simulink model "EMR_vehicle_model"  (R2023a)
settings: Solver=VariableStepAuto  StartTime=0.0  StopTime=10.0  RelTol=1e-3
values from neighbouring files (symbols this model uses):
  A_f = 2    [parameter_definiciton.m]
  air_dens = 1.22521    [parameter_definiciton.m]
  angle_road = atan(slope_road/100)    [parameter_definiciton.m]
  C_d = 0.35    [parameter_definiciton.m]
  f_r = 0.017    [parameter_definiciton.m]
  g = 9.8    [parameter_definiciton.m]
  m_v = 1000    [parameter_definiciton.m]
  wind_speed = 0    [parameter_definiciton.m]
libraries: simulink x1
settings Model: Creator=citcea  LastModifiedBy=citcea

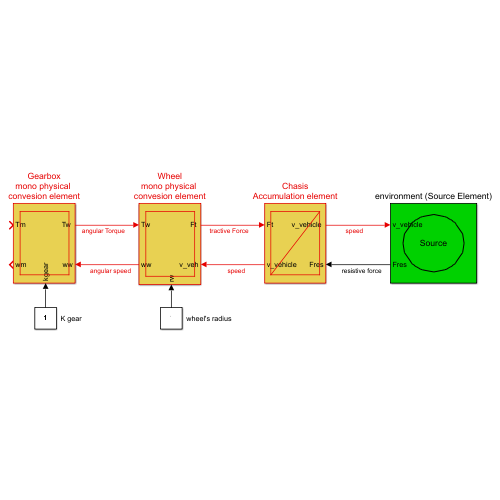
[thumbnail: Simulink's stored preview of the top-level diagram]
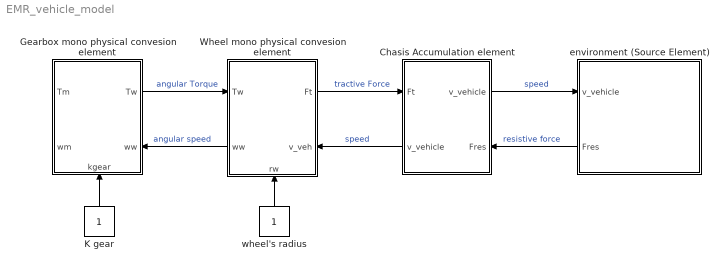
== system EMR_vehicle_model ==
  Chasis Accumulation element : Subsystem  mask(CM){}
      settings: LibrarySourceBlock=simulink/REM/EA  PortSchema="{\"entries\":[{\"content\":{\"sides\":[{\"content\":{\"connectorIds\":[\"In1\",\"Out2\"]},\"type\":\"ConnectorPlacement.EquallySpacedRectSide\",\"uuid\":\"dba36025-b2f5-41cb-9761-d1287a9766e1\"},{\"content\":{\"connectorIds\":[\"Out1\",\"In2\"],\"side\":\"RIGHT\"},\"type\":\"ConnectorPlacement.EquallySpacedRectSide\",\"uuid\":\"3ae5e504-7b8f-4c00-bc0d-c89eccd87070\"},{\"content\":{\"side\":\"TOP\"},\"type\":\"ConnectorPlacement.EquallySpacedRectSide\",\"uuid\":\"a4c04bb5-f94e-4b5c-882d-2c32a11c6b0c\"}]},\"type\":\"ConnectorPlacement.EquallySpacedConnector\",\"uuid\":\"0c2b765b-f129-495b-87a6-76b6e14d78ec\"}],\"packageUris\":[\"http://schema.mathworks.com/mf0/Connector/R2020b\"],\"version\":\"1.0\"}"
      mask Display: plot(0,0,100,100,[10,10,90,90,10],[90,10,10,90,90], [10,90],[10,90])
  Gearbox mono physical convesion element : Subsystem  mask(Hacheur){}
      settings: LibrarySourceBlock=simulink/REM/EC Elec  PortSchema="{\"entries\":[{\"content\":{\"sides\":[{\"content\":{\"connectorIds\":[\"In1\",\"Out2\"]},\"type\":\"ConnectorPlacement.EquallySpacedRectSide\",\"uuid\":\"add9fadb-0fb4-43ab-a2d0-7727804eb2c0\"},{\"content\":{\"connectorIds\":[\"Out1\",\"In3\"],\"side\":\"RIGHT\"},\"type\":\"ConnectorPlacement.EquallySpacedRectSide\",\"uuid\":\"87b3f5c0-7da9-421a-ae8a-66afee038ab7\"},{\"content\":{\"side\":\"TOP\"},\"type\":\"ConnectorPlacement.EquallySpacedRectSide\",\"uuid\":\"1a4f8f42-25ac-452e-8ff7-6a9f16bc9892\"},{\"content\":{\"connectorIds\":[\"In2\"],\"side\":\"BOTTOM\"},\"type\":\"ConnectorPlacement.EquallySpacedRectSide\",\"uuid\":\"62447f74-8a92-4f32-9436-8aa69c6390a6\"}]},\"type\":\"ConnectorPlacement.EquallySpacedConnector\",\"uuid\":\"bc965109-6171-440e-b0fd-d7c986fb98ff\"}],\"packageUris\":[\"http://schema.mathworks.com/mf0/Connector/R2020b\"],\"version\":\"1.0\"}"
      mask Display: plot(0,0,100,100,[10,10,90,90,10],[90,10,10,90,90])
  K gear : Constant
  Wheel mono physical convesion element : Subsystem  mask(Hacheur){}
      settings: LibrarySourceBlock=simulink/REM/EC Elec  PortSchema="{\"entries\":[{\"content\":{\"sides\":[{\"content\":{\"connectorIds\":[\"In1\",\"Out2\"]},\"type\":\"ConnectorPlacement.EquallySpacedRectSide\",\"uuid\":\"add9fadb-0fb4-43ab-a2d0-7727804eb2c0\"},{\"content\":{\"connectorIds\":[\"Out1\",\"In3\"],\"side\":\"RIGHT\"},\"type\":\"ConnectorPlacement.EquallySpacedRectSide\",\"uuid\":\"87b3f5c0-7da9-421a-ae8a-66afee038ab7\"},{\"content\":{\"side\":\"TOP\"},\"type\":\"ConnectorPlacement.EquallySpacedRectSide\",\"uuid\":\"1a4f8f42-25ac-452e-8ff7-6a9f16bc9892\"},{\"content\":{\"connectorIds\":[\"In2\"],\"side\":\"BOTTOM\"},\"type\":\"ConnectorPlacement.EquallySpacedRectSide\",\"uuid\":\"cb138da9-d7db-4398-93fc-4ebc55a3031f\"}]},\"type\":\"ConnectorPlacement.EquallySpacedConnector\",\"uuid\":\"bc965109-6171-440e-b0fd-d7c986fb98ff\"}],\"packageUris\":[\"http://schema.mathworks.com/mf0/Connector/R2020b\"],\"version\":\"1.0\"}"
      mask Display: plot(0,0,100,100,[10,10,90,90,10],[90,10,10,90,90])
  environment (Source Element) : Subsystem
      settings: LibrarySourceBlock=simulink/REM/SE  PortSchema="{\"entries\":[{\"content\":{\"sides\":[{\"content\":{\"connectorIds\":[\"In1\",\"Out1\"]},\"type\":\"ConnectorPlacement.EquallySpacedRectSide\",\"uuid\":\"5172ac9f-d5c1-4cd8-b96a-59474b42a5b1\"},{\"content\":{\"side\":\"RIGHT\"},\"type\":\"ConnectorPlacement.EquallySpacedRectSide\",\"uuid\":\"2f1e5561-012a-4a4f-9618-a2ea7815b4bb\"},{\"content\":{\"side\":\"TOP\"},\"type\":\"ConnectorPlacement.EquallySpacedRectSide\",\"uuid\":\"04863bbd-e2a6-484f-917f-c8a12d5dbdba\"}]},\"type\":\"ConnectorPlacement.EquallySpacedConnector\",\"uuid\":\"d1a021b9-616a-4321-9b00-fb5e0223e97f\"}],\"packageUris\":[\"http://schema.mathworks.com/mf0/Connector/R2020b\"],\"version\":\"1.0\"}"
      mask Display:
      | plot(0,0,100,100, 1.2*[50,57.68,60.77,63.08,64.97,66.58,68,69.26,70.4, 	71.42,72.36,78.28,80,78.28,72.36,71.42,70.4, 	69.26,68,66.58,64.97,63.08,60.77,57.68,50,42.32, 	39.23,36.92,35.03,33.42,32,30.74,29.6,28.58, 	27.64,21.72,20,21.72,27.64,28.58,29.6,30.74,32, 	33.42,35.03,36.92,39.23,42.32,50]-10, 1.2*[20,21,22,23,24,25,26,27,28,29,30,40,50,60,70,71,72, 	73,74,75,76,77,78,79,80,79,78,77,76,75,74,73,72, 	71,70,60,50,40,30,29,28,27,26,25,24,23,22,21,20]-10)
      | disp('Source')
  wheel's radius : Constant
  wires:
  Chasis Accumulation element/1("v_vehicle ") -> environment (Source Element)/1(v_vehicle)  "speed"
  environment (Source Element)/1(Fres) -> Chasis Accumulation element/2(Fres)  "resistive force"
  Wheel mono physical convesion element/1("Ft ") -> Chasis Accumulation element/1(Ft)  "tractive Force"
  Chasis Accumulation element/2(v_vehicle) -> Wheel mono physical convesion element/3(v_veh)  "speed"
  wheel's radius/1 -> Wheel mono physical convesion element/2(rw)
  Gearbox mono physical convesion element/1("Tw ") -> Wheel mono physical convesion element/1(Tw)  "angular Torque"
  Wheel mono physical convesion element/2(ww) -> Gearbox mono physical convesion element/3(ww)  "angular speed"
  K gear/1 -> Gearbox mono physical convesion element/2(kgear)

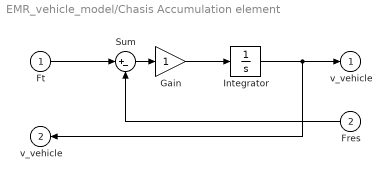
== system EMR_vehicle_model/Chasis Accumulation element ==
  Ft : Inport
  Fres : Inport  Port=2
  Gain : Gain
  Integrator : Integrator
  Sum : Sum  Inputs=|+-
  "v_vehicle " : Outport  InitialOutput=0
  v_vehicle : Outport  Port=2  InitialOutput=0
  wires:
  Gain/1 -> Integrator/1
  Sum/1 -> Gain/1
  Integrator/1 -> v_vehicle/1, "v_vehicle "/1
  Ft/1 -> Sum/1
  Fres/1 -> Sum/2

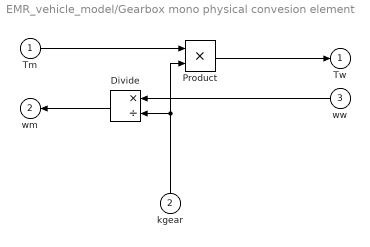
== system EMR_vehicle_model/Gearbox mono physical convesion element ==
  Tm : Inport
  kgear : Inport  Port=2
  ww : Inport  Port=3
  Divide : Product  Inputs=*/
  Product : Product
  "Tw " : Outport  InitialOutput=0
  wm : Outport  Port=2  InitialOutput=0
  wires:
  Divide/1 -> wm/1
  kgear/1 -> Divide/2, Product/2
  ww/1 -> Divide/1
  Product/1 -> "Tw "/1
  Tm/1 -> Product/1

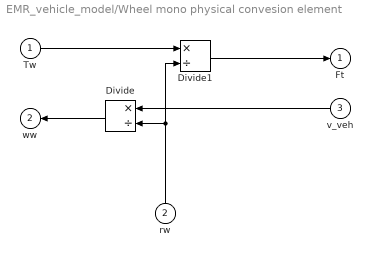
== system EMR_vehicle_model/Wheel mono physical convesion element ==
  Tw : Inport
  rw : Inport  Port=2
  v_veh : Inport  Port=3
  Divide : Product  Inputs=*/
  Divide1 : Product  Inputs=*/
  "Ft " : Outport  InitialOutput=0
  ww : Outport  Port=2  InitialOutput=0
  wires:
  Divide/1 -> ww/1
  v_veh/1 -> Divide/1
  rw/1 -> Divide1/2, Divide/2
  Divide1/1 -> "Ft "/1
  Tw/1 -> Divide1/1

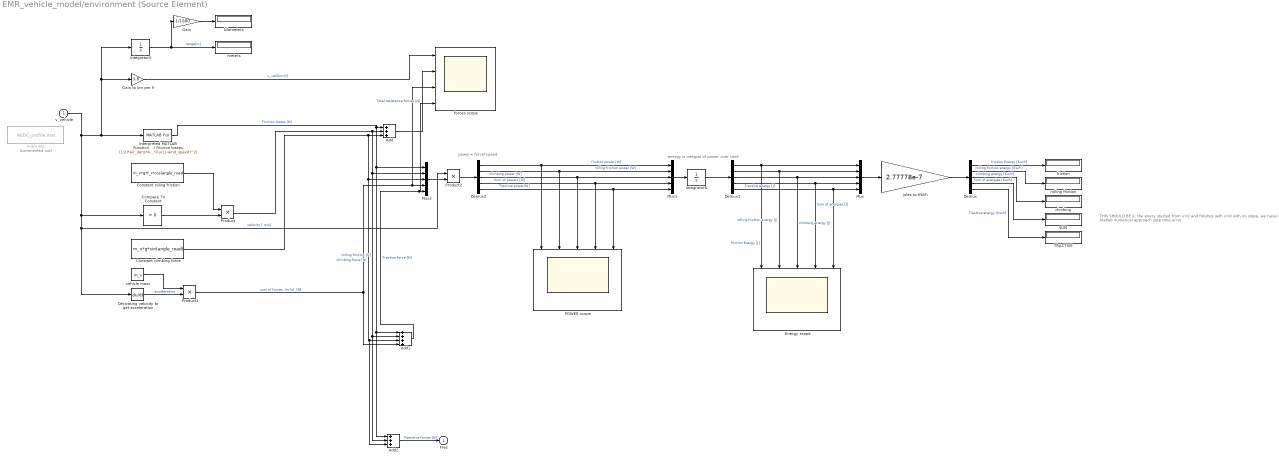
== system EMR_vehicle_model/environment (Source Element) ==
  note: energy is integral of power over time
  note: power= force*speed
  note: THIS SHOULD BE 0, the enery started from v=0 and finishes with v=0 with no slope. we have a matlab numerical approach step time error
  v_vehicle : Inport
  Add : Sum  Inputs=+++
  Add1 : Sum  Inputs=++++
  Add2 : Sum  Inputs=+++
  Compare To Constant : simulink/Logic and Bit Operations/Compare To Constant  relop=>  const=0  OutDataTypeStr=boolean
  Constant climbing force : Constant  Value=m_v*g*sin(angle_road)
  Constant roling friction : Constant  Value=m_v*g*f_r*cos(angle_road)
  Demux : Demux  Outputs=5
  Demux1 : Demux  Outputs=5
  Demux2 : Demux  Outputs=5
  Derivating velocity to get acceleration : Derivative
  Energy scope : Scope  NumInputPorts=5
  From File : FromFile  Commented=on  FileName=NEDC_profile.mat  SampleTime=0
  Gain : Gain  Gain=1/1000
  Gain to km per h : Gain  Gain=3.6
  Integrator5 : Integrator
  Integrator6 : Integrator
  Interpreted MATLAB Function Aerodinamical friccion losses : MATLABFcn  MATLABFcn=(1/2)*air_dens*A_f*C_d*((u(1)-wind_speed)^2)
  Mux : Mux  Inputs=5
  Mux1 : Mux  Inputs=5
  Mux2 : Mux  Inputs=5
  POWER scope : Scope  NumInputPorts=5
  Product : Product
  Product1 : Product
  Product2 : Product
  "SUM " : Display
  TRACTIVE : Display
  climbing : Display
  forces scope : Scope  NumInputPorts=4
  friction : Display
  jules to KW/h : Gain  Gain=2.77778e-7
  kilometers : Display
  meters : Display
  "rolling friction " : Display
  vehicle mass : Constant  Value=m_v
  Fres : Outport  InitialOutput=0
  wires:
  Add2/1 -> Fres/1  "Resistive forces [N]"
  Gain/1 -> kilometers/1
  v_vehicle/1 -> Derivating velocity to get acceleration/1, Product2/1, Compare To Constant/1, Integrator5/1, Gain to km per h/1, Interpreted MATLAB Function Aerodinamical friccion losses/1  "velocity [ m/s]"
  Add1/1 -> forces scope/4, Mux2/5  "Traction force [N]"
  Demux2/2 -> Mux1/2, POWER scope/2  "rolling friction power [W]"
  Integrator5/1 -> Gain/1, meters/1  "range[m]"
  Demux/3 -> climbing/1  "climbing energy [Kw/h]"
  Constant roling friction/1 -> Product/1
  Mux2/1 -> Product2/2
  Gain to km per h/1 -> forces scope/1  "v_veh[km/h]"
  Demux1/3 -> Energy scope/3, Mux/3  "climbing energy [J]"
  Compare To Constant/1 -> Product/2
  Demux2/5 -> Mux1/5, POWER scope/5  "Tractive power[W]"
  Mux1/1 -> Integrator6/1
  Product2/1 -> Demux2/1
  jules to KW/h/1 -> Demux/1
  Demux1/2 -> Energy scope/2, Mux/2  "rolling friction energy [J]"
  Demux/2 -> "rolling friction "/1  "rolling friction energy [Kw/h]"
  Demux2/1 -> Mux1/1, POWER scope/1  "friction power [W]"
  Constant climbing force/1 -> Add2/3, Add1/3, Mux2/3, Add/3  "climbing force [N]"
  Add/1 -> forces scope/2  "Total resistance forces [N]"
  Interpreted MATLAB Function Aerodinamical friccion losses/1 -> Add1/1, Add2/1, Mux2/1, Add/1  "Friction losses [N]"
  Demux2/4 -> Mux1/4, POWER scope/4  "Sum of powers [W]"
  Demux1/4 -> Energy scope/4, Mux/4  "Sum of energies [J]"
  Demux1/1 -> Mux/1, Energy scope/1  "friction Energy [J]"
  Demux1/5 -> Energy scope/5, Mux/5  "Tractive energy [J]"
  Derivating velocity to get acceleration/1 -> Product1/2  "acceleration"
  Integrator6/1 -> Demux1/1
  Mux/1 -> jules to KW/h/1
  Demux2/3 -> Mux1/3, POWER scope/3  "climbing power [W]"
  Product/1 -> Add2/2, Add1/2, Mux2/2, Add/2  "rolling friction [N]"
  Demux/5 -> TRACTIVE/1  "Tractive energy [Kw/h]"
  vehicle mass/1 -> Product1/1
  Demux/4 -> "SUM "/1  "Sum of energies [Kw/h]"
  Demux/1 -> friction/1  "friction Energy [Kw/h]"
  Product1/1 -> Mux2/4, forces scope/3, Add1/4  "sum of forces  (m*a)  [N]"
